simulink model "UAM_Acutuator"  (R2024b)
settings: Solver=VariableStepAuto  StartTime=0.0  StopTime=10.0  RelTol=1e-3
undefined symbols (not defined in the file): contact, env, F, iniRoll, initPitch, iniYaw, Light, MIL, minPWM, uavParam, vIni, xGround, yGround, zGround
libraries: matrix_library x8, robotcorelib x4, sharedtransform x3, aerolibasang x2, aerolibwind2 x2, shared6dof x1, aerolibadyn x1
(part 2 of 2)

== system UAM_Acutuator/Force and Moments/Aerodynamic Forces/Compute Body Frame Forces and Moments/Wind frame F& M/Longitudinal Channel/Cm ==
  alpha : Inport
  De : Inport  Port=2
  p,q,r : Inport  Port=3
  Airspeed : Inport  Port=4
  Cm0 : Constant  Value=uavParam.aero.Cm0
      settings: AttributesFormatString=%<Value>
  CmDe : Constant  Value=uavParam.aero.CmDe
      settings: AttributesFormatString=%<Value>
  Cma : Constant  Value=uavParam.aero.Cma
      settings: AttributesFormatString=%<Value>
  Lift due to pitch rate : Subsystem
  Product1 : Product  Inputs=**  SaturateOnIntegerOverflow=on  OutDataTypeStr=Inherit: Same as first input
  Product4 : Product  SaturateOnIntegerOverflow=on  OutDataTypeStr=Inherit: Same as first input
  Sum : Sum  Inputs=+++++  SaturateOnIntegerOverflow=on
  Cm : Outport  VectorParamsAs1DForOutWhenUnconnected=off
  wires:
  Lift due to pitch rate/1(Cmq) -> Sum/5  "cmq"
  p,q,r/1 -> Lift due to pitch rate/1(p,q,r)
  Product1/1 -> Sum/3  "cmde"
  Product4/1 -> Sum/2  "cma"
  Sum/1 -> Cm/1  "total"
  De/1 -> Product1/2
  CmDe/1 -> Product1/1
  Cma/1 -> Product4/1
  Cm0/1 -> Sum/1  "cm0"
  Airspeed/1 -> Lift due to pitch rate/2(Airspeed)
  alpha/1 -> Product4/2

== system UAM_Acutuator/Force and Moments/Aerodynamic Forces/Compute Body Frame Forces and Moments/Wind frame F& M/Lateral Channel/CY/roll factors ==
  p,q,r : Inport
  Airspeed : Inport  Port=2
  Constant : Constant  Value=uavParam.aero.CYp
      settings: AttributesFormatString=%<Value>
  Constant1 : Constant  Value=uavParam.aero.CYr
      settings: AttributesFormatString=%<Value>
  Get p : Selector  InputPortWidth=3  IndexOptions=Index vector (dialog)  Indices=1  OutputSizes=[(-2)]
  Get r : Selector  InputPortWidth=3  IndexOptions=Index vector (dialog)  Indices=3  OutputSizes=[(-2)]
  Product : Product  SaturateOnIntegerOverflow=on  OutDataTypeStr=Inherit: Same as first input
  Product1 : Product  SaturateOnIntegerOverflow=on  OutDataTypeStr=Inherit: Same as first input
  Subsystem : Subsystem
  roll rate fact : Subsystem
  CYp : Outport  VectorParamsAs1DForOutWhenUnconnected=off
  CYr : Outport  Port=2  VectorParamsAs1DForOutWhenUnconnected=off
  wires:
  Get r/1 -> Subsystem/1(r)
  p,q,r/1 -> Get r/1, Get p/1
  Get p/1 -> roll rate fact/1(p)
  Airspeed/1 -> Subsystem/2(Airspeed), roll rate fact/2(Airspeed)
  Subsystem/1(Yaw Rate Fac) -> Product1/2
  Constant1/1 -> Product1/1
  roll rate fact/1(Roll Rate Fac) -> Product/2
  Constant/1 -> Product/1
  Product1/1 -> CYr/1
  Product/1 -> CYp/1

== system UAM_Acutuator/Force and Moments/Aerodynamic Forces/Compute Body Frame Forces and Moments/Wind frame F& M/Lateral Channel/Cl/roll factors ==
  p,q,r : Inport
  Airspeed : Inport  Port=2
  Constant : Constant  Value=uavParam.aero.Clp
      settings: AttributesFormatString=%<Value>
  Constant1 : Constant  Value=uavParam.aero.Clr
      settings: AttributesFormatString=%<Value>
  Get p : Selector  InputPortWidth=3  IndexOptions=Index vector (dialog)  Indices=1  OutputSizes=[(-2)]
  Get r : Selector  InputPortWidth=3  IndexOptions=Index vector (dialog)  Indices=3  OutputSizes=[(-2)]
  Product : Product  SaturateOnIntegerOverflow=on  OutDataTypeStr=Inherit: Same as first input
  Product1 : Product  SaturateOnIntegerOverflow=on  OutDataTypeStr=Inherit: Same as first input
  roll rate fact : Subsystem
  yaw rate fact : Subsystem
  Clp : Outport  VectorParamsAs1DForOutWhenUnconnected=off
  Clr : Outport  Port=2  VectorParamsAs1DForOutWhenUnconnected=off
  wires:
  Get r/1 -> yaw rate fact/1(r)
  p,q,r/1 -> Get r/1, Get p/1
  Get p/1 -> roll rate fact/1(p)
  Airspeed/1 -> yaw rate fact/2(Airspeed), roll rate fact/2(Airspeed)
  yaw rate fact/1(Yaw Rate Fac) -> Product1/2
  Constant1/1 -> Product1/1
  roll rate fact/1(Roll Rate Fac) -> Product/2
  Constant/1 -> Product/1
  Product1/1 -> Clr/1
  Product/1 -> Clp/1

== system UAM_Acutuator/Force and Moments/Aerodynamic Forces/Compute Body Frame Forces and Moments/Wind frame F& M/Lateral Channel/Cn/yaw factors ==
  p,q,r : Inport
  Airspeed : Inport  Port=2
  Constant : Constant  Value=uavParam.aero.Cnp
      settings: AttributesFormatString=%<Value>
  Constant1 : Constant  Value=uavParam.aero.Cnr
      settings: AttributesFormatString=%<Value>
  Get p : Selector  InputPortWidth=3  IndexOptions=Index vector (dialog)  Indices=1  OutputSizes=[(-2)]
  Get r : Selector  InputPortWidth=3  IndexOptions=Index vector (dialog)  Indices=3  OutputSizes=[(-2)]
  Product : Product  SaturateOnIntegerOverflow=on  OutDataTypeStr=Inherit: Same as first input
  Product1 : Product  SaturateOnIntegerOverflow=on  OutDataTypeStr=Inherit: Same as first input
  roll rate fact : Subsystem
  yaw rate fact1 : Subsystem
  Cnp : Outport  VectorParamsAs1DForOutWhenUnconnected=off
  Cnr : Outport  Port=2  VectorParamsAs1DForOutWhenUnconnected=off
  wires:
  Airspeed/1 -> yaw rate fact1/2(Airspeed), roll rate fact/2(Airspeed)
  Get r/1 -> yaw rate fact1/1(r)
  p,q,r/1 -> Get r/1, Get p/1
  Get p/1 -> roll rate fact/1(p)
  roll rate fact/1(Roll Rate Fac) -> Product/2
  Constant/1 -> Product/1
  yaw rate fact1/1(Yaw Rate Fac) -> Product1/2
  Constant1/1 -> Product1/1
  Product1/1 -> Cnr/1
  Product/1 -> Cnp/1

== system UAM_Acutuator/Force and Moments/Aerodynamic Forces/Compute Body Frame Forces and Moments/Wind frame F& M/Longitudinal Channel/CL/Lift due to pitch rate ==
  p,q,r : Inport
  Airspeed : Inport  Port=2
  Constant : Constant  Value=uavParam.aero.CLq
      settings: AttributesFormatString=%<Value>
  Get q : Selector  InputPortWidth=3  IndexOptions=Index vector (dialog)  Indices=2  OutputSizes=[(-2)]
  Product : Product  SaturateOnIntegerOverflow=on  OutDataTypeStr=Inherit: Same as first input
  pitch rate factor : Subsystem
  CLq : Outport  VectorParamsAs1DForOutWhenUnconnected=off
  wires:
  Airspeed/1 -> pitch rate factor/2(Airspeed)
  Get q/1 -> pitch rate factor/1(q)
  p,q,r/1 -> Get q/1
  Product/1 -> CLq/1
  pitch rate factor/1(Pitch Rate Fac) -> Product/2
  Constant/1 -> Product/1

== system UAM_Acutuator/Force and Moments/Aerodynamic Forces/Compute Body Frame Forces and Moments/Wind frame F& M/Longitudinal Channel/Cm/Lift due to pitch rate ==
  p,q,r : Inport
  Airspeed : Inport  Port=2
  Constant : Constant  Value=uavParam.aero.Cmq
      settings: AttributesFormatString=%<Value>
  Get q : Selector  InputPortWidth=3  IndexOptions=Index vector (dialog)  Indices=2  OutputSizes=[(-2)]
  Product : Product  SaturateOnIntegerOverflow=on  OutDataTypeStr=Inherit: Same as first input
  pitch rate factor : Subsystem
  Cmq : Outport  VectorParamsAs1DForOutWhenUnconnected=off
  wires:
  Airspeed/1 -> pitch rate factor/2(Airspeed)
  Get q/1 -> pitch rate factor/1(q)
  p,q,r/1 -> Get q/1
  Product/1 -> Cmq/1
  pitch rate factor/1(Pitch Rate Fac) -> Product/2
  Constant/1 -> Product/1

== system UAM_Acutuator/Force and Moments/Aerodynamic Forces/Compute Body Frame Forces and Moments/Wind frame F& M/Lateral Channel/CY/roll factors/Subsystem ==
  r : Inport
  Airspeed : Inport  Port=2
  Cmq3 : Constant
      settings: AttributesFormatString=%<Value>
  Cmq4 : Constant  Value=uavParam.geom.b
      settings: AttributesFormatString=%<Value>
  Gain : Gain  Gain=2
  Product1 : Product  Inputs=***/  SaturateOnIntegerOverflow=on  OutDataTypeStr=Inherit: Same as first input
  Saturation : Saturate  UpperLimit=inf  LowerLimit=0.1
      settings: AttributesFormatString="[%<LowerLimit>  %<UpperLimit>]"
  Yaw Rate Fac : Outport  VectorParamsAs1DForOutWhenUnconnected=off
  wires:
  Saturation/1 -> Gain/1
  Cmq4/1 -> Product1/3
  Airspeed/1 -> Saturation/1
  Gain/1 -> Product1/4
  Cmq3/1 -> Product1/2
  Product1/1 -> Yaw Rate Fac/1
  r/1 -> Product1/1

== system UAM_Acutuator/Force and Moments/Aerodynamic Forces/Compute Body Frame Forces and Moments/Wind frame F& M/Lateral Channel/CY/roll factors/roll rate fact ==
  p : Inport
  Airspeed : Inport  Port=2
  Cmq1 : Constant
      settings: AttributesFormatString=%<Value>
  Cmq2 : Constant  Value=uavParam.geom.b
      settings: AttributesFormatString=%<Value>
  Gain : Gain  Gain=2
  Product : Product  Inputs=***/  SaturateOnIntegerOverflow=on  OutDataTypeStr=Inherit: Same as first input
  Saturation : Saturate  UpperLimit=inf  LowerLimit=0.1
      settings: AttributesFormatString="[%<LowerLimit>  %<UpperLimit>]"
  Roll Rate Fac : Outport  VectorParamsAs1DForOutWhenUnconnected=off
  wires:
  Airspeed/1 -> Saturation/1
  Cmq2/1 -> Product/3
  Cmq1/1 -> Product/2
  p/1 -> Product/1
  Product/1 -> Roll Rate Fac/1
  Saturation/1 -> Gain/1
  Gain/1 -> Product/4

== system UAM_Acutuator/Force and Moments/Aerodynamic Forces/Compute Body Frame Forces and Moments/Wind frame F& M/Lateral Channel/Cl/roll factors/roll rate fact ==
  p : Inport
  Airspeed : Inport  Port=2
  Cmq1 : Constant  Value=.5
      settings: AttributesFormatString=%<Value>
  Cmq2 : Constant  Value=uavParam.geom.b
      settings: AttributesFormatString=%<Value>
  Product : Product  Inputs=***/  SaturateOnIntegerOverflow=on  OutDataTypeStr=Inherit: Same as first input
  Saturation : Saturate  UpperLimit=inf  LowerLimit=0.1
      settings: AttributesFormatString="[%<LowerLimit>  %<UpperLimit>]"
  Roll Rate Fac : Outport  VectorParamsAs1DForOutWhenUnconnected=off
  wires:
  Saturation/1 -> Product/4
  Airspeed/1 -> Saturation/1
  Cmq2/1 -> Product/3
  Cmq1/1 -> Product/2
  p/1 -> Product/1
  Product/1 -> Roll Rate Fac/1

== system UAM_Acutuator/Force and Moments/Aerodynamic Forces/Compute Body Frame Forces and Moments/Wind frame F& M/Lateral Channel/Cl/roll factors/yaw rate fact ==
  r : Inport
  Airspeed : Inport  Port=2
  Cmq3 : Constant  Value=.5
      settings: AttributesFormatString=%<Value>
  Cmq4 : Constant  Value=uavParam.geom.b
      settings: AttributesFormatString=%<Value>
  Product1 : Product  Inputs=***/  SaturateOnIntegerOverflow=on  OutDataTypeStr=Inherit: Same as first input
  Saturation : Saturate  UpperLimit=inf  LowerLimit=0.1
      settings: AttributesFormatString="[%<LowerLimit>  %<UpperLimit>]"
  Yaw Rate Fac : Outport
  wires:
  Airspeed/1 -> Saturation/1
  Saturation/1 -> Product1/4
  r/1 -> Product1/1
  Product1/1 -> Yaw Rate Fac/1
  Cmq4/1 -> Product1/3
  Cmq3/1 -> Product1/2

== system UAM_Acutuator/Force and Moments/Aerodynamic Forces/Compute Body Frame Forces and Moments/Wind frame F& M/Lateral Channel/Cn/yaw factors/roll rate fact ==
  p : Inport
  Airspeed : Inport  Port=2
  Cmq1 : Constant  Value=.5
      settings: AttributesFormatString=%<Value>
  Cmq2 : Constant  Value=uavParam.geom.b
      settings: AttributesFormatString=%<Value>
  Product : Product  Inputs=***/  SaturateOnIntegerOverflow=on  OutDataTypeStr=Inherit: Same as first input
  Saturation : Saturate  UpperLimit=inf  LowerLimit=0.1
      settings: AttributesFormatString="[%<LowerLimit>  %<UpperLimit>]"
  Roll Rate Fac : Outport  VectorParamsAs1DForOutWhenUnconnected=off
  wires:
  Saturation/1 -> Product/4
  Airspeed/1 -> Saturation/1
  Cmq2/1 -> Product/3
  Cmq1/1 -> Product/2
  p/1 -> Product/1
  Product/1 -> Roll Rate Fac/1

== system UAM_Acutuator/Force and Moments/Aerodynamic Forces/Compute Body Frame Forces and Moments/Wind frame F& M/Lateral Channel/Cn/yaw factors/yaw rate fact1 ==
  r : Inport
  Airspeed : Inport  Port=2
  Cmq3 : Constant  Value=.5
      settings: AttributesFormatString=%<Value>
  Cmq4 : Constant  Value=uavParam.geom.b
      settings: AttributesFormatString=%<Value>
  Product1 : Product  Inputs=***/  SaturateOnIntegerOverflow=on  OutDataTypeStr=Inherit: Same as first input
  Saturation : Saturate  UpperLimit=inf  LowerLimit=0.1
      settings: AttributesFormatString="[%<LowerLimit>  %<UpperLimit>]"
  Yaw Rate Fac : Outport
  wires:
  Airspeed/1 -> Saturation/1
  Saturation/1 -> Product1/4
  r/1 -> Product1/1
  Product1/1 -> Yaw Rate Fac/1
  Cmq4/1 -> Product1/3
  Cmq3/1 -> Product1/2

== system UAM_Acutuator/Force and Moments/Aerodynamic Forces/Compute Body Frame Forces and Moments/Wind frame F& M/Longitudinal Channel/CL/Lift due to pitch rate/pitch rate factor ==
  q : Inport
  Airspeed : Inport  Port=2
  Cmq2 : Constant  Value=uavParam.geom.c
      settings: AttributesFormatString=%<Value>
  Gain : Gain  Gain=2
  Product : Product  Inputs=**/  SaturateOnIntegerOverflow=on  OutDataTypeStr=Inherit: Same as first input
  Saturation : Saturate  UpperLimit=inf  LowerLimit=0.1
      settings: AttributesFormatString="[%<LowerLimit>  %<UpperLimit>]"
  Pitch Rate Fac : Outport  VectorParamsAs1DForOutWhenUnconnected=off
  wires:
  Cmq2/1 -> Product/2
  Airspeed/1 -> Saturation/1
  q/1 -> Product/1
  Product/1 -> Pitch Rate Fac/1
  Saturation/1 -> Gain/1
  Gain/1 -> Product/3

== system UAM_Acutuator/Force and Moments/Aerodynamic Forces/Compute Body Frame Forces and Moments/Wind frame F& M/Longitudinal Channel/Cm/Lift due to pitch rate/pitch rate factor ==
  q : Inport
  Airspeed : Inport  Port=2
  Cmq2 : Constant  Value=uavParam.geom.c
      settings: AttributesFormatString=%<Value>
  Gain : Gain  Gain=2
  Product : Product  Inputs=**/  SaturateOnIntegerOverflow=on  OutDataTypeStr=Inherit: Same as first input
  Saturation : Saturate  UpperLimit=inf  LowerLimit=0.1
      settings: AttributesFormatString="[%<LowerLimit>  %<UpperLimit>]"
  Pitch Rate Fac : Outport  VectorParamsAs1DForOutWhenUnconnected=off
  wires:
  Cmq2/1 -> Product/2
  Airspeed/1 -> Saturation/1
  q/1 -> Product/1
  Product/1 -> Pitch Rate Fac/1
  Saturation/1 -> Gain/1
  Gain/1 -> Product/3

== matlab function UAM_Acutuator/Feedback/MATLAB Function1 ==
  data: vxyz input; course output; gndSpeed output
function [course, gndSpeed] = fcn(vxyz)

vx = vxyz(1);
vy = vxyz(2);
course = atan2(vy, vx);
gndSpeed = norm([vx vy 0]);

== matlab function UAM_Acutuator/Ground Truth Bus/MATLAB Function1 ==
  data: vxyz input; course output; gndSpeed output
function [course, gndSpeed] = fcn(vxyz)

vx = vxyz(1);
vy = vxyz(2);
course = atan2(vy, vx);
gndSpeed = norm([vx vy 0]);
